simulink model "armacdm"  (R2018a)
settings: Solver=VariableStepAuto  StartTime=0.0  StopTime=10  RelTol=1e-3
values from neighbouring files (symbols this model uses):
  A = cosh(vl)    [kpavanmatlab.m]
libraries: powerlib x6
settings Model: Creator=pc  LastModifiedBy=pc

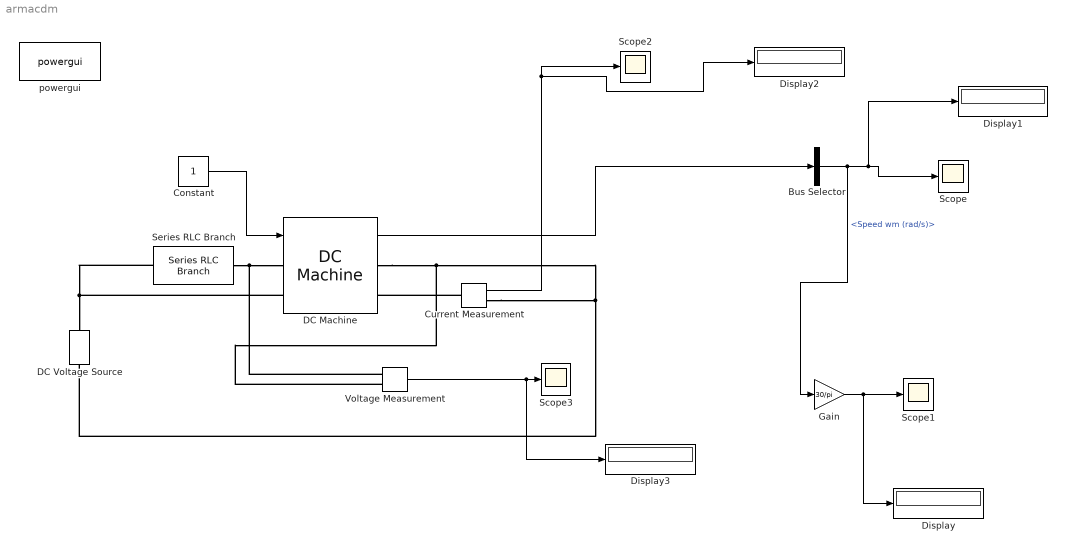
== system armacdm ==
  Bus Selector : BusSelector  OutputSignals=Speed wm (rad/s)
  Constant : Constant
  Current Measurement : powerlib/Measurements/Current Measurement  PhasorSimulation=off  OutputType=Complex  PSBequivalent=0
  DC Machine : powerlib/Machines/DC Machine  PresetModel=No  MechanicalLoad=Torque TL  FieldType=Wound  ShowDetailedParameters=on  MeasurementBus=off  RLa="[ 0.6  0.012]"  RLf="[ 240  120]"  Laf=1.8  MachineConstant=Torque constant (N.m/A)  Ke=1.8  Kt=1.8  J=1  Bm=0  Tf=0  w0=1  Ifinit=1  TsPowergui=0  TsBlock=-1
  DC Voltage Source : powerlib/Electrical Sources/DC Voltage Source  Amplitude=240  Measurements=None
  Display{,1..3} (4 alike) : Display
  Gain : Gain  Gain=30/pi
  Scope{,1..3} (4 alike) : Scope
  Series RLC Branch : powerlib/Elements/Series RLC Branch  LConnTagsString=__new0  RConnTagsString=__new0  BranchType=R  Resistance=200  Inductance=1e-3  SetiL0=off  InitialCurrent=0  Capacitance=1e-6  Setx0=off  InitialVoltage=0  Measurements=None
  Voltage Measurement : powerlib/Measurements/Voltage Measurement  PhasorSimulation=off  OutputType=Complex  PSBequivalent=0
  powergui : powerlib/powergui  Priority=1  SimulationMode=Continuous  SampleTime=50e-6  frequency=60  Iterations=50  frequencyindice=0  Pbase=100e6  ErrMax=1e-4  UnitsV=kV  UnitsW=MW  buscounter=0  FunctionMessages=off  echomessages=off  EnableUseOfTLC=off  CurrentSourceSwitches=off  DisableSnubberDevices=off  DisableRonSwitches=off  DisableVfSwitches=off  DisplayEquations=off  SolverType=Tustin/Backward Euler (TBE)  Interpol=off  ExternalGateDelay=off  methode=off  Ts=100  x0status=blocks  SPID=on  SwTol=0  HookPort=off  RestoreLinks=warning  ResistiveCurrentMeasurement=off  Frange=[0:2:500]  Ylog=off  Xlog=on  ShowGrid=off  save=off  variable=ZData  structure=0  ZoomFFT=off  StartTime=0.0  cycles=1  DisplayStyle=1  fundamental=60  FreqAxis=off  MaxFrequency=1000  frequencyindicesteady=1  RmsSteady=1  display=off
  wires:
  Current Measurement/1 -> Display2/1, Scope2/1
  DC Machine/1 -> Bus Selector/1
  Gain/1 -> Display/1, Scope1/1
  Bus Selector/1 -> Gain/1, Display1/1, Scope/1  "<Speed wm (rad/s)>"
  Constant/1 -> DC Machine/1
  Voltage Measurement/1 -> Display3/1, Scope3/1
  connections:
  DC Voltage Source/LConn1 -- Voltage Measurement/LConn2 -- DC Machine/RConn1 -- Current Measurement/RConn1
  Series RLC Branch/LConn1 -- DC Machine/LConn2 -- DC Voltage Source/RConn1
  Current Measurement/LConn1 -- DC Machine/RConn2
  Series RLC Branch/RConn1 -- Voltage Measurement/LConn1 -- DC Machine/LConn1
